simulink library "LRLM"  (R2021a)
settings: Solver=VariableStepAuto  StartTime=0.0  StopTime=10.0  RelTol=1e-3
libraries: simulink x2
settings Model: Creator=Sai229  LastModifiedBy=Sai229

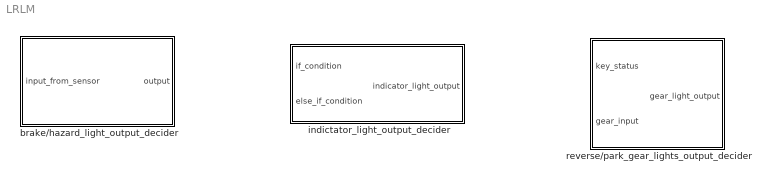
== system LRLM ==
  brake/hazard_light_output_decider : Subsystem  mask(Brake and Hazard Light Output decider){}
      mask help: This system decides the output of brake and hazard lights, whether they are on or off. Connect the brake sensor or the hazard switch sensor to the input and based on the input the output port will turn on or turn off brake lights or hazard lights
  indictator_light_output_decider : Subsystem  mask(Indicator lights output decider){}
      mask help: This system decides the output of indicator lights (left and right indicators) whether they are on or off. Connect the signal to if_condition input when you want the indicator lights to blink. Connect the signal to else_if_condition input when you want the indicator lights to remain in off condition. The output of this system can be connected to merge blocks.
  reverse/park_gear_lights_output_decider : Subsystem  mask(Reverse/Park gear lights output decider){gear_option=Neutral}
      mask prompts: gear_option "Enter the gear option"
      mask help: This system decides the output of the reverse gear lights and park gear lights. Connect the key status to key_input and gear sensor input to gear_option button. Connect the output to the gear lights
      mask TypeOptions gear_option: Neutral | Drive | Park | Reverse

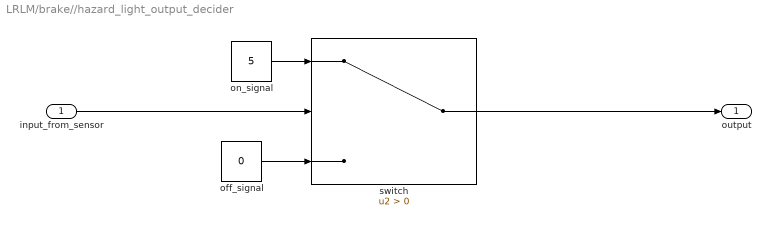
== system LRLM/brake//hazard_light_output_decider ==
  input_from_sensor : Inport
  off_signal : Constant  Value=0  VectorParams1D=off  SampleTime=-1
  on_signal : Constant  Value=5  VectorParams1D=off  SampleTime=-1
  switch : Switch  Criteria=u2 > Threshold
  output : Outport
  wires:
  on_signal/1 -> switch/1
  off_signal/1 -> switch/3
  switch/1 -> output/1
  input_from_sensor/1 -> switch/2

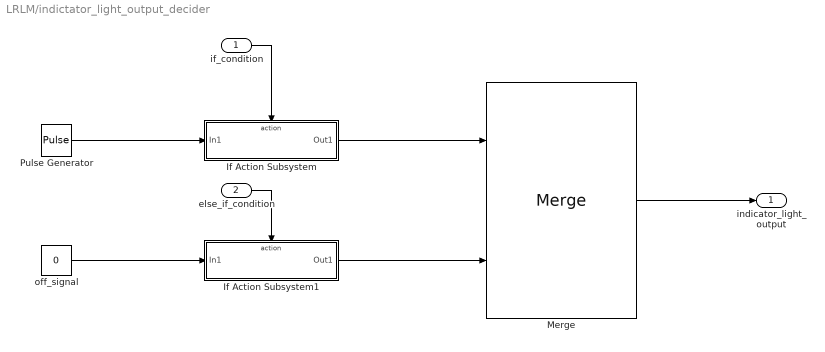
== system LRLM/indictator_light_output_decider ==
  if_condition : Inport
  else_if_condition : Inport  Port=2
  If Action Subsystem : Subsystem  TreatAsAtomicUnit=on
  If Action Subsystem1 : Subsystem  TreatAsAtomicUnit=on
  Merge : Merge
  Pulse Generator : DiscretePulseGenerator  PulseType=Time based  Amplitude=5  Period=0.1  PulseWidth=50
  off_signal : Constant  Value=0
  indicator_light_output : Outport
  wires:
  else_if_condition/1 -> If Action Subsystem1/Action
  Pulse Generator/1 -> If Action Subsystem/1(In1)
  off_signal/1 -> If Action Subsystem1/1(In1)
  if_condition/1 -> If Action Subsystem/Action
  If Action Subsystem/1(Out1) -> Merge/1
  If Action Subsystem1/1(Out1) -> Merge/2
  Merge/1 -> indicator_light_output/1

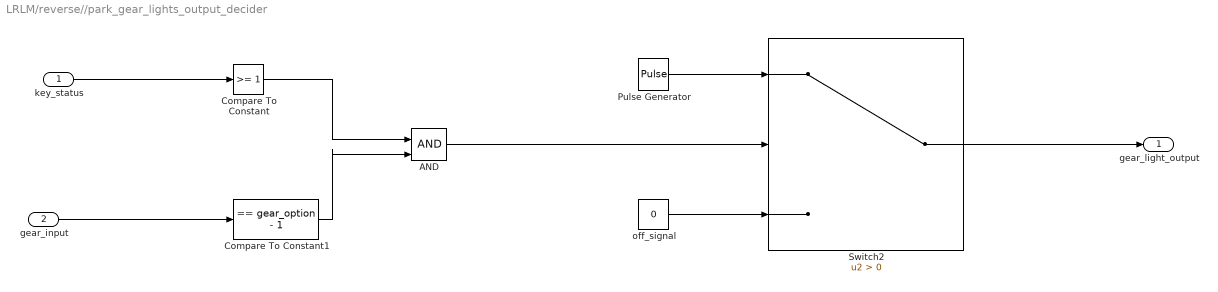
== system LRLM/reverse//park_gear_lights_output_decider ==
  key_status : Inport
  gear_input : Inport  Port=2
  AND : Logic  IconShape=distinctive  AllPortsSameDT=off  OutDataTypeStr=boolean
  Compare To Constant : simulink/Logic and Bit Operations/Compare To Constant  relop=>=  const=1  OutDataTypeStr=boolean
  Compare To Constant1 : simulink/Logic and Bit Operations/Compare To Constant  relop===  const=gear_option - 1  OutDataTypeStr=boolean
  Pulse Generator : DiscretePulseGenerator  PulseType=Time based  Amplitude=5  Period=0.1  PulseWidth=50
  Switch2 : Switch  Criteria=u2 > Threshold
  off_signal : Constant  Value=0
  gear_light_output : Outport
  wires:
  Compare To Constant1/1 -> AND/2
  Compare To Constant/1 -> AND/1
  off_signal/1 -> Switch2/3
  AND/1 -> Switch2/2
  Pulse Generator/1 -> Switch2/1
  gear_input/1 -> Compare To Constant1/1
  key_status/1 -> Compare To Constant/1
  Switch2/1 -> gear_light_output/1

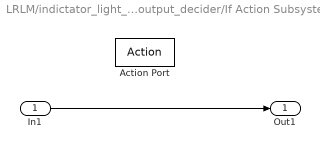
== system LRLM/indictator_light_output_decider/If Action Subsystem ==
  In1 : Inport
  Action Port : ActionPort
  Out1 : Outport
  wires:
  In1/1 -> Out1/1

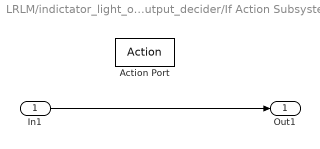
== system LRLM/indictator_light_output_decider/If Action Subsystem1 ==
  In1 : Inport
  Action Port : ActionPort
  Out1 : Outport
  wires:
  In1/1 -> Out1/1
